simulink model "Sim_Induct_Harmon"  (R2019a)
settings: Solver=FixedStepAuto  StartTime=0.0  StopTime=sim_time  FixedStep=1e-6  MaxStep=1e-4  RelTol=1e-3
values from neighbouring files (symbols this model uses):
  J = 0.0025    [motor_parameters.mat]
  Laq = 0.001    [motor_parameters.mat]
  Lse = 0.001    [motor_parameters.mat]
  Ra = 2.08    [motor_parameters.mat]
  Rse = 5.7    [motor_parameters.mat]
  SEIP4 = [-14.225 -12.275 -10.725 -9.725 -9.1 -8.6 -8.075 -7.65 -7.2 -6.85 -6.492 -6.135 ... (45 elements, 1x45)]    [motor_parameters.mat]
  SEVP4 = [-160 -155 -150 -145 -140 -135 -130 -125 -120 -115 -110 -105 ... (45 elements, 1x45)]    [motor_parameters.mat]
  sim_off = sim_on    [double_load.m]    (also in fourfold_load.m; individual_load.m; triple_load.m)
  sim_on = 50*ones(1,28)    [double_load.m]    (also in fourfold_load.m; individual_load.m; triple_load.m)
  wm0 = 0    [motor_parameters.mat]
  wmo = 157.079632679    [motor_parameters.mat]
undefined symbols (not defined in the file or in its folder): C21, C22, C23, C24, L41, L42, L43, L44, L61, L62, L63, L64, R, R21, R22, R23, R24, R31, R32, R33, R34, R41, R42, R43, R44, R51, R52, R53, R54, R61, R62, R63, R64, R71, R72, R73, R74, Valpha5, Valpha6
libraries: powerlib x225, simulink x72
(part 2 of 3)

== system Sim_Induct_Harmon/ON_OFF_26 ==
  Clock8 : Clock
  Compare To Constant5 : simulink/Logic and Bit Operations/Compare To Constant  relop=>=  const=sim_on(26)  OutDataTypeStr=boolean
  Compare To Constat6 : simulink/Logic and Bit Operations/Compare To Constant  relop=<=  const=sim_off(26)  OutDataTypeStr=boolean
  OFF5 : powerlib/Power Electronics/Ideal Switch  Ron=0.001  Lon=0  IC=0  Rs=1e5  Cs=inf  Measurements=off
      settings: SourceProductName=Simscape Electrical
  ON5 : powerlib/Power Electronics/Ideal Switch  Ron=0.001  Lon=0  IC=0  Rs=1e5  Cs=inf  Measurements=off
      settings: SourceProductName=Simscape Electrical
  Conn1 : PMIOPort  Side=Left
  Conn2 : PMIOPort  Port=2  Side=Right
  wires:
  Clock8/1 -> Compare To Constat6/1, Compare To Constant5/1
  Compare To Constat6/1 -> OFF5/1
  Compare To Constant5/1 -> ON5/1
  connections:
  ON5/RConn1 -- OFF5/LConn1
  OFF5/RConn1 -- Conn2/RConn1
  ON5/LConn1 -- Conn1/RConn1

== system Sim_Induct_Harmon/ON_OFF_27 ==
  Clock8 : Clock
  Compare To Constant5 : simulink/Logic and Bit Operations/Compare To Constant  relop=>=  const=sim_on(27)  OutDataTypeStr=boolean
  Compare To Constat6 : simulink/Logic and Bit Operations/Compare To Constant  relop=<=  const=sim_off(27)  OutDataTypeStr=boolean
  OFF5 : powerlib/Power Electronics/Ideal Switch  Ron=0.001  Lon=0  IC=0  Rs=1e5  Cs=inf  Measurements=off
      settings: SourceProductName=Simscape Electrical
  ON5 : powerlib/Power Electronics/Ideal Switch  Ron=0.001  Lon=0  IC=0  Rs=1e5  Cs=inf  Measurements=off
      settings: SourceProductName=Simscape Electrical
  Conn1 : PMIOPort  Side=Left
  Conn2 : PMIOPort  Port=2  Side=Right
  wires:
  Clock8/1 -> Compare To Constat6/1, Compare To Constant5/1
  Compare To Constat6/1 -> OFF5/1
  Compare To Constant5/1 -> ON5/1
  connections:
  ON5/RConn1 -- OFF5/LConn1
  OFF5/RConn1 -- Conn2/RConn1
  ON5/LConn1 -- Conn1/RConn1

== system Sim_Induct_Harmon/ON_OFF_28 ==
  Clock8 : Clock
  Compare To Constant5 : simulink/Logic and Bit Operations/Compare To Constant  relop=>=  const=sim_on(28)  OutDataTypeStr=boolean
  Compare To Constat6 : simulink/Logic and Bit Operations/Compare To Constant  relop=<=  const=sim_off(28)  OutDataTypeStr=boolean
  OFF5 : powerlib/Power Electronics/Ideal Switch  Ron=0.001  Lon=0  IC=0  Rs=1e5  Cs=inf  Measurements=off
      settings: SourceProductName=Simscape Electrical
  ON5 : powerlib/Power Electronics/Ideal Switch  Ron=0.001  Lon=0  IC=0  Rs=1e5  Cs=inf  Measurements=off
      settings: SourceProductName=Simscape Electrical
  Conn1 : PMIOPort  Side=Left
  Conn2 : PMIOPort  Port=2  Side=Right
  wires:
  Clock8/1 -> Compare To Constat6/1, Compare To Constant5/1
  Compare To Constat6/1 -> OFF5/1
  Compare To Constant5/1 -> ON5/1
  connections:
  ON5/RConn1 -- OFF5/LConn1
  OFF5/RConn1 -- Conn2/RConn1
  ON5/LConn1 -- Conn1/RConn1

== system Sim_Induct_Harmon/ON_OFF_3 ==
  Clock1 : Clock
  Clock2 : Clock
  Clock3 : Clock
  Compare To Constant : simulink/Logic and Bit Operations/Compare To Constant  relop=>=  const=sim_on(3)  OutDataTypeStr=boolean
  Compare To Constant1 : simulink/Logic and Bit Operations/Compare To Constant  relop=>=  const=sim_off(3)  OutDataTypeStr=boolean
  Compare To Constant2 : simulink/Logic and Bit Operations/Compare To Constant  relop=>=  const=sim_on(3)  OutDataTypeStr=boolean
  Constant : Constant  Value=0
  Constant1 : Constant  Value=0
  Ideal Switch : powerlib/Power Electronics/Ideal Switch  Ron=0.001  Lon=0  IC=0  Rs=1e5  Cs=inf  Measurements=off
      settings: SourceProductName=Simscape Electrical
  Switch : Switch
  Switch1 : Switch
  Conn1 : PMIOPort  Side=Left
  Conn2 : PMIOPort  Port=2  Side=Left
  tag scope: tensao_3=global
  wires:
  Switch1/1 -> [tensao_3]
  Constant/1 -> Switch/3
  Switch/1 -> Switch1/3
  Clock1/1 -> Compare To Constant/1
  Clock2/1 -> Compare To Constant1/1
  Compare To Constant1/1 -> Switch1/2
  [fonte_tensao] -> Switch/1
  Constant1/1 -> Switch1/1
  Compare To Constant/1 -> Switch/2
  Clock3/1 -> Compare To Constant2/1
  Compare To Constant2/1 -> Ideal Switch/1
  connections:
  Conn1/RConn1 -- Ideal Switch/LConn1
  Ideal Switch/RConn1 -- Conn2/RConn1

== system Sim_Induct_Harmon/ON_OFF_4 ==
  Clock1 : Clock
  Clock2 : Clock
  Clock3 : Clock
  Compare To Constant : simulink/Logic and Bit Operations/Compare To Constant  relop=>=  const=sim_on(4)  OutDataTypeStr=boolean
  Compare To Constant1 : simulink/Logic and Bit Operations/Compare To Constant  relop=>=  const=sim_off(4)  OutDataTypeStr=boolean
  Compare To Constant2 : simulink/Logic and Bit Operations/Compare To Constant  relop=>=  const=sim_on(4)  OutDataTypeStr=boolean
  Constant : Constant  Value=0
  Constant1 : Constant  Value=0
  Ideal Switch : powerlib/Power Electronics/Ideal Switch  Ron=0.001  Lon=0  IC=0  Rs=1e5  Cs=inf  Measurements=off
      settings: SourceProductName=Simscape Electrical
  Switch : Switch
  Switch1 : Switch
  Conn1 : PMIOPort  Side=Left
  Conn2 : PMIOPort  Port=2  Side=Left
  tag scope: tensao_4=global
  wires:
  Switch1/1 -> [tensao_4]
  Constant/1 -> Switch/3
  Switch/1 -> Switch1/3
  Clock1/1 -> Compare To Constant/1
  Clock2/1 -> Compare To Constant1/1
  Compare To Constant1/1 -> Switch1/2
  [fonte_tensao] -> Switch/1
  Constant1/1 -> Switch1/1
  Compare To Constant/1 -> Switch/2
  Clock3/1 -> Compare To Constant2/1
  Compare To Constant2/1 -> Ideal Switch/1
  connections:
  Conn1/RConn1 -- Ideal Switch/LConn1
  Ideal Switch/RConn1 -- Conn2/RConn1

== system Sim_Induct_Harmon/ON_OFF_5 ==
  Clock1 : Clock
  Compare To Constant1 : simulink/Logic and Bit Operations/Compare To Constant  relop=>=  const=sim_on(5)  OutDataTypeStr=boolean
  Compare To Constat1 : simulink/Logic and Bit Operations/Compare To Constant  relop=<=  const=sim_off(5)  OutDataTypeStr=boolean
  OFF1 : powerlib/Power Electronics/Ideal Switch  Ron=0.001  Lon=0  IC=0  Rs=1e5  Cs=inf  Measurements=off
      settings: SourceProductName=Simscape Electrical
  ON1 : powerlib/Power Electronics/Ideal Switch  Ron=0.001  Lon=0  IC=0  Rs=1e5  Cs=inf  Measurements=off
      settings: SourceProductName=Simscape Electrical
  Conn1 : PMIOPort  Side=Left
  Conn2 : PMIOPort  Port=2  Side=Right
  wires:
  Compare To Constat1/1 -> OFF1/1
  Compare To Constant1/1 -> ON1/1
  Clock1/1 -> Compare To Constat1/1, Compare To Constant1/1
  connections:
  ON1/RConn1 -- OFF1/LConn1
  Conn1/RConn1 -- ON1/LConn1
  OFF1/RConn1 -- Conn2/RConn1

== system Sim_Induct_Harmon/ON_OFF_6 ==
  Clock1 : Clock
  Compare To Constant1 : simulink/Logic and Bit Operations/Compare To Constant  relop=>=  const=sim_on(6)  OutDataTypeStr=boolean
  Compare To Constat1 : simulink/Logic and Bit Operations/Compare To Constant  relop=<=  const=sim_off(6)  OutDataTypeStr=boolean
  OFF1 : powerlib/Power Electronics/Ideal Switch  Ron=0.001  Lon=0  IC=0  Rs=1e5  Cs=inf  Measurements=off
      settings: SourceProductName=Simscape Electrical
  ON1 : powerlib/Power Electronics/Ideal Switch  Ron=0.001  Lon=0  IC=0  Rs=1e5  Cs=inf  Measurements=off
      settings: SourceProductName=Simscape Electrical
  Conn1 : PMIOPort  Side=Left
  Conn2 : PMIOPort  Port=2  Side=Right
  wires:
  Compare To Constat1/1 -> OFF1/1
  Compare To Constant1/1 -> ON1/1
  Clock1/1 -> Compare To Constat1/1, Compare To Constant1/1
  connections:
  ON1/RConn1 -- OFF1/LConn1
  Conn1/RConn1 -- ON1/LConn1
  OFF1/RConn1 -- Conn2/RConn1

== system Sim_Induct_Harmon/ON_OFF_7 ==
  Clock1 : Clock
  Compare To Constant1 : simulink/Logic and Bit Operations/Compare To Constant  relop=>=  const=sim_on(7)  OutDataTypeStr=boolean
  Compare To Constat1 : simulink/Logic and Bit Operations/Compare To Constant  relop=<=  const=sim_off(7)  OutDataTypeStr=boolean
  OFF1 : powerlib/Power Electronics/Ideal Switch  Ron=0.001  Lon=0  IC=0  Rs=1e5  Cs=inf  Measurements=off
      settings: SourceProductName=Simscape Electrical
  ON1 : powerlib/Power Electronics/Ideal Switch  Ron=0.001  Lon=0  IC=0  Rs=1e5  Cs=inf  Measurements=off
      settings: SourceProductName=Simscape Electrical
  Conn1 : PMIOPort  Side=Left
  Conn2 : PMIOPort  Port=2  Side=Right
  wires:
  Compare To Constat1/1 -> OFF1/1
  Compare To Constant1/1 -> ON1/1
  Clock1/1 -> Compare To Constat1/1, Compare To Constant1/1
  connections:
  ON1/RConn1 -- OFF1/LConn1
  Conn1/RConn1 -- ON1/LConn1
  OFF1/RConn1 -- Conn2/RConn1

== system Sim_Induct_Harmon/ON_OFF_8 ==
  Clock1 : Clock
  Compare To Constant1 : simulink/Logic and Bit Operations/Compare To Constant  relop=>=  const=sim_on(8)  OutDataTypeStr=boolean
  Compare To Constat1 : simulink/Logic and Bit Operations/Compare To Constant  relop=<=  const=sim_off(8)  OutDataTypeStr=boolean
  OFF1 : powerlib/Power Electronics/Ideal Switch  Ron=0.001  Lon=0  IC=0  Rs=1e5  Cs=inf  Measurements=off
      settings: SourceProductName=Simscape Electrical
  ON1 : powerlib/Power Electronics/Ideal Switch  Ron=0.001  Lon=0  IC=0  Rs=1e5  Cs=inf  Measurements=off
      settings: SourceProductName=Simscape Electrical
  Conn1 : PMIOPort  Side=Left
  Conn2 : PMIOPort  Port=2  Side=Right
  wires:
  Compare To Constat1/1 -> OFF1/1
  Compare To Constant1/1 -> ON1/1
  Clock1/1 -> Compare To Constat1/1, Compare To Constant1/1
  connections:
  ON1/RConn1 -- OFF1/LConn1
  Conn1/RConn1 -- ON1/LConn1
  OFF1/RConn1 -- Conn2/RConn1

== system Sim_Induct_Harmon/ON_OFF_9 ==
  Clock4 : Clock
  Compare To Constant2 : simulink/Logic and Bit Operations/Compare To Constant  relop=>=  const=sim_on(9)  OutDataTypeStr=boolean
  Compare To Constat3 : simulink/Logic and Bit Operations/Compare To Constant  relop=<=  const=sim_off(9)  OutDataTypeStr=boolean
  OFF2 : powerlib/Power Electronics/Ideal Switch  Ron=0.001  Lon=0  IC=0  Rs=1e5  Cs=inf  Measurements=off
      settings: SourceProductName=Simscape Electrical
  ON2 : powerlib/Power Electronics/Ideal Switch  Ron=0.001  Lon=0  IC=0  Rs=1e5  Cs=inf  Measurements=off
      settings: SourceProductName=Simscape Electrical
  Conn1 : PMIOPort  Side=Left
  Conn2 : PMIOPort  Port=2  Side=Right
  wires:
  Compare To Constant2/1 -> ON2/1
  Compare To Constat3/1 -> OFF2/1
  Clock4/1 -> Compare To Constat3/1, Compare To Constant2/1
  connections:
  OFF2/RConn1 -- Conn2/RConn1
  ON2/RConn1 -- OFF2/LConn1
  ON2/LConn1 -- Conn1/RConn1

== system Sim_Induct_Harmon/RL_1 ==
  note: LOAD
  Scope : Scope
  Scope1 : Scope
  Series RLC Branch : powerlib/Elements/Series RLC Branch  LConnTagsString=__new0  RConnTagsString=__new0  BranchType=R  Resistance=R41  Inductance=1e-3  SetiL0=off  InitialCurrent=0  Capacitance=1e-6  Setx0=off  InitialVoltage=0  Measurements=None
      settings: SourceProductName=Simscape Electrical
  Series RLC Branch1 : powerlib/Elements/Series RLC Branch  LConnTagsString=__new0  RConnTagsString=__new0  BranchType=L  Resistance=1  Inductance=L41  SetiL0=off  InitialCurrent=0  Capacitance=1e-6  Setx0=off  InitialVoltage=0  Measurements=None
      settings: SourceProductName=Simscape Electrical
  To Workspace1 : ToWorkspace  VariableName=corrente_rl_1  SampleTime=-1
  To Workspace4 : ToWorkspace  VariableName=tensao_rl_1  SampleTime=-1
  V_Load : powerlib/Measurements/Voltage Measurement  PhasorSimulation=off  OutputType=Complex  PSBequivalent=0
      settings: SourceProductName=Simscape Electrical
  i_Load : powerlib/Measurements/Current Measurement  Tag=PoWeRsYsTeMmEaSuReMeNt  PhasorSimulation=off  OutputType=Magnitude  PSBequivalent=0
      settings: SourceProductName=Simscape Electrical
  Conn1 : PMIOPort  Side=Left
  Conn2 : PMIOPort  Port=2  Side=Left
  wires:
  V_Load/1 -> To Workspace4/1, Scope/1
  i_Load/1 -> To Workspace1/1, Scope1/1
  connections:
  Series RLC Branch/LConn1 -- V_Load/LConn1 -- i_Load/RConn1
  Conn1/RConn1 -- i_Load/LConn1
  V_Load/LConn2 -- Conn2/RConn1 -- Series RLC Branch1/RConn1
  Series RLC Branch1/LConn1 -- Series RLC Branch/RConn1

== system Sim_Induct_Harmon/RL_2 ==
  note: LOAD
  Scope : Scope
  Scope1 : Scope
  Series RLC Branch : powerlib/Elements/Series RLC Branch  LConnTagsString=__new0  RConnTagsString=__new0  BranchType=R  Resistance=R42  Inductance=1e-3  SetiL0=off  InitialCurrent=0  Capacitance=1e-6  Setx0=off  InitialVoltage=0  Measurements=None
      settings: SourceProductName=Simscape Electrical
  Series RLC Branch1 : powerlib/Elements/Series RLC Branch  LConnTagsString=__new0  RConnTagsString=__new0  BranchType=L  Resistance=1  Inductance=L42  SetiL0=off  InitialCurrent=0  Capacitance=1e-6  Setx0=off  InitialVoltage=0  Measurements=None
      settings: SourceProductName=Simscape Electrical
  To Workspace1 : ToWorkspace  VariableName=corrente_rl_2  SampleTime=-1
  To Workspace4 : ToWorkspace  VariableName=tensao_rl_2  SampleTime=-1
  V_Load : powerlib/Measurements/Voltage Measurement  PhasorSimulation=off  OutputType=Complex  PSBequivalent=0
      settings: SourceProductName=Simscape Electrical
  i_Load : powerlib/Measurements/Current Measurement  Tag=PoWeRsYsTeMmEaSuReMeNt  PhasorSimulation=off  OutputType=Magnitude  PSBequivalent=0
      settings: SourceProductName=Simscape Electrical
  Conn1 : PMIOPort  Side=Left
  Conn2 : PMIOPort  Port=2  Side=Left
  wires:
  V_Load/1 -> To Workspace4/1, Scope/1
  i_Load/1 -> To Workspace1/1, Scope1/1
  connections:
  Series RLC Branch/LConn1 -- V_Load/LConn1 -- i_Load/RConn1
  Conn1/RConn1 -- i_Load/LConn1
  V_Load/LConn2 -- Conn2/RConn1 -- Series RLC Branch1/RConn1
  Series RLC Branch1/LConn1 -- Series RLC Branch/RConn1

== system Sim_Induct_Harmon/RL_3 ==
  note: LOAD
  Scope : Scope
  Scope1 : Scope
  Series RLC Branch : powerlib/Elements/Series RLC Branch  LConnTagsString=__new0  RConnTagsString=__new0  BranchType=R  Resistance=R43  Inductance=1e-3  SetiL0=off  InitialCurrent=0  Capacitance=1e-6  Setx0=off  InitialVoltage=0  Measurements=None
      settings: SourceProductName=Simscape Electrical
  Series RLC Branch1 : powerlib/Elements/Series RLC Branch  LConnTagsString=__new0  RConnTagsString=__new0  BranchType=L  Resistance=1  Inductance=L43  SetiL0=off  InitialCurrent=0  Capacitance=1e-6  Setx0=off  InitialVoltage=0  Measurements=None
      settings: SourceProductName=Simscape Electrical
  To Workspace1 : ToWorkspace  VariableName=corrente_rl_3  SampleTime=-1
  To Workspace4 : ToWorkspace  VariableName=tensao_rl_3  SampleTime=-1
  V_Load : powerlib/Measurements/Voltage Measurement  PhasorSimulation=off  OutputType=Complex  PSBequivalent=0
      settings: SourceProductName=Simscape Electrical
  i_Load : powerlib/Measurements/Current Measurement  Tag=PoWeRsYsTeMmEaSuReMeNt  PhasorSimulation=off  OutputType=Magnitude  PSBequivalent=0
      settings: SourceProductName=Simscape Electrical
  Conn1 : PMIOPort  Side=Left
  Conn2 : PMIOPort  Port=2  Side=Left
  wires:
  V_Load/1 -> To Workspace4/1, Scope/1
  i_Load/1 -> To Workspace1/1, Scope1/1
  connections:
  Series RLC Branch/LConn1 -- V_Load/LConn1 -- i_Load/RConn1
  Conn1/RConn1 -- i_Load/LConn1
  V_Load/LConn2 -- Conn2/RConn1 -- Series RLC Branch1/RConn1
  Series RLC Branch1/LConn1 -- Series RLC Branch/RConn1

== system Sim_Induct_Harmon/RL_4 ==
  note: LOAD
  Scope : Scope
  Scope1 : Scope
  Series RLC Branch : powerlib/Elements/Series RLC Branch  LConnTagsString=__new0  RConnTagsString=__new0  BranchType=R  Resistance=R44  Inductance=1e-3  SetiL0=off  InitialCurrent=0  Capacitance=1e-6  Setx0=off  InitialVoltage=0  Measurements=None
      settings: SourceProductName=Simscape Electrical
  Series RLC Branch1 : powerlib/Elements/Series RLC Branch  LConnTagsString=__new0  RConnTagsString=__new0  BranchType=L  Resistance=1  Inductance=L44  SetiL0=off  InitialCurrent=0  Capacitance=1e-6  Setx0=off  InitialVoltage=0  Measurements=None
      settings: SourceProductName=Simscape Electrical
  To Workspace1 : ToWorkspace  VariableName=corrente_rl_4  SampleTime=-1
  To Workspace4 : ToWorkspace  VariableName=tensao_rl_4  SampleTime=-1
  V_Load : powerlib/Measurements/Voltage Measurement  PhasorSimulation=off  OutputType=Complex  PSBequivalent=0
      settings: SourceProductName=Simscape Electrical
  i_Load : powerlib/Measurements/Current Measurement  Tag=PoWeRsYsTeMmEaSuReMeNt  PhasorSimulation=off  OutputType=Magnitude  PSBequivalent=0
      settings: SourceProductName=Simscape Electrical
  Conn1 : PMIOPort  Side=Left
  Conn2 : PMIOPort  Port=2  Side=Left
  wires:
  V_Load/1 -> To Workspace4/1, Scope/1
  i_Load/1 -> To Workspace1/1, Scope1/1
  connections:
  Series RLC Branch/LConn1 -- V_Load/LConn1 -- i_Load/RConn1
  Conn1/RConn1 -- i_Load/LConn1
  V_Load/LConn2 -- Conn2/RConn1 -- Series RLC Branch1/RConn1
  Series RLC Branch1/LConn1 -- Series RLC Branch/RConn1

== system Sim_Induct_Harmon/R_1 ==
  note: LOAD
  Scope : Scope
  Scope1 : Scope
  Series RLC Branch : powerlib/Elements/Series RLC Branch  LConnTagsString=__new0  RConnTagsString=__new0  BranchType=R  Resistance=R31  Inductance=1e-3  SetiL0=off  InitialCurrent=0  Capacitance=1e-6  Setx0=off  InitialVoltage=0  Measurements=None
      settings: SourceProductName=Simscape Electrical
  To Workspace1 : ToWorkspace  VariableName=corrente_r_1  SampleTime=-1
  To Workspace4 : ToWorkspace  VariableName=tensao_r_1  SampleTime=-1
  V_Load : powerlib/Measurements/Voltage Measurement  PhasorSimulation=off  OutputType=Complex  PSBequivalent=0
      settings: SourceProductName=Simscape Electrical
  i_Load : powerlib/Measurements/Current Measurement  Tag=PoWeRsYsTeMmEaSuReMeNt  PhasorSimulation=off  OutputType=Magnitude  PSBequivalent=0
      settings: SourceProductName=Simscape Electrical
  Conn1 : PMIOPort  Side=Left
  Conn2 : PMIOPort  Port=2  Side=Left
  wires:
  V_Load/1 -> To Workspace4/1, Scope/1
  i_Load/1 -> To Workspace1/1, Scope1/1
  connections:
  Series RLC Branch/LConn1 -- V_Load/LConn1 -- i_Load/RConn1
  Series RLC Branch/RConn1 -- V_Load/LConn2 -- Conn2/RConn1
  Conn1/RConn1 -- i_Load/LConn1

== system Sim_Induct_Harmon/R_2 ==
  note: LOAD
  Scope : Scope
  Scope1 : Scope
  Series RLC Branch : powerlib/Elements/Series RLC Branch  LConnTagsString=__new0  RConnTagsString=__new0  BranchType=R  Resistance=R32  Inductance=1e-3  SetiL0=off  InitialCurrent=0  Capacitance=1e-6  Setx0=off  InitialVoltage=0  Measurements=None
      settings: SourceProductName=Simscape Electrical
  To Workspace1 : ToWorkspace  VariableName=corrente_r_2  SampleTime=-1
  To Workspace4 : ToWorkspace  VariableName=tensao_r_2  SampleTime=-1
  V_Load : powerlib/Measurements/Voltage Measurement  PhasorSimulation=off  OutputType=Complex  PSBequivalent=0
      settings: SourceProductName=Simscape Electrical
  i_Load : powerlib/Measurements/Current Measurement  Tag=PoWeRsYsTeMmEaSuReMeNt  PhasorSimulation=off  OutputType=Magnitude  PSBequivalent=0
      settings: SourceProductName=Simscape Electrical
  Conn1 : PMIOPort  Side=Left
  Conn2 : PMIOPort  Port=2  Side=Left
  wires:
  V_Load/1 -> To Workspace4/1, Scope/1
  i_Load/1 -> To Workspace1/1, Scope1/1
  connections:
  Series RLC Branch/LConn1 -- V_Load/LConn1 -- i_Load/RConn1
  Series RLC Branch/RConn1 -- V_Load/LConn2 -- Conn2/RConn1
  Conn1/RConn1 -- i_Load/LConn1

== system Sim_Induct_Harmon/R_3 ==
  note: LOAD
  Scope : Scope
  Scope1 : Scope
  Series RLC Branch : powerlib/Elements/Series RLC Branch  LConnTagsString=__new0  RConnTagsString=__new0  BranchType=R  Resistance=R33  Inductance=1e-3  SetiL0=off  InitialCurrent=0  Capacitance=1e-6  Setx0=off  InitialVoltage=0  Measurements=None
      settings: SourceProductName=Simscape Electrical
  To Workspace1 : ToWorkspace  VariableName=corrente_r_3  SampleTime=-1
  To Workspace4 : ToWorkspace  VariableName=tensao_r_3  SampleTime=-1
  V_Load : powerlib/Measurements/Voltage Measurement  PhasorSimulation=off  OutputType=Complex  PSBequivalent=0
      settings: SourceProductName=Simscape Electrical
  i_Load : powerlib/Measurements/Current Measurement  Tag=PoWeRsYsTeMmEaSuReMeNt  PhasorSimulation=off  OutputType=Magnitude  PSBequivalent=0
      settings: SourceProductName=Simscape Electrical
  Conn1 : PMIOPort  Side=Left
  Conn2 : PMIOPort  Port=2  Side=Left
  wires:
  V_Load/1 -> To Workspace4/1, Scope/1
  i_Load/1 -> To Workspace1/1, Scope1/1
  connections:
  Series RLC Branch/LConn1 -- V_Load/LConn1 -- i_Load/RConn1
  Series RLC Branch/RConn1 -- V_Load/LConn2 -- Conn2/RConn1
  Conn1/RConn1 -- i_Load/LConn1

== system Sim_Induct_Harmon/R_4 ==
  note: LOAD
  Scope : Scope
  Scope1 : Scope
  Series RLC Branch : powerlib/Elements/Series RLC Branch  LConnTagsString=__new0  RConnTagsString=__new0  BranchType=R  Resistance=R34  Inductance=1e-3  SetiL0=off  InitialCurrent=0  Capacitance=1e-6  Setx0=off  InitialVoltage=0  Measurements=None
      settings: SourceProductName=Simscape Electrical
  To Workspace1 : ToWorkspace  VariableName=corrente_r_4  SampleTime=-1
  To Workspace4 : ToWorkspace  VariableName=tensao_r_4  SampleTime=-1
  V_Load : powerlib/Measurements/Voltage Measurement  PhasorSimulation=off  OutputType=Complex  PSBequivalent=0
      settings: SourceProductName=Simscape Electrical
  i_Load : powerlib/Measurements/Current Measurement  Tag=PoWeRsYsTeMmEaSuReMeNt  PhasorSimulation=off  OutputType=Magnitude  PSBequivalent=0
      settings: SourceProductName=Simscape Electrical
  Conn1 : PMIOPort  Side=Left
  Conn2 : PMIOPort  Port=2  Side=Left
  wires:
  V_Load/1 -> To Workspace4/1, Scope/1
  i_Load/1 -> To Workspace1/1, Scope1/1
  connections:
  Series RLC Branch/LConn1 -- V_Load/LConn1 -- i_Load/RConn1
  Series RLC Branch/RConn1 -- V_Load/LConn2 -- Conn2/RConn1
  Conn1/RConn1 -- i_Load/LConn1

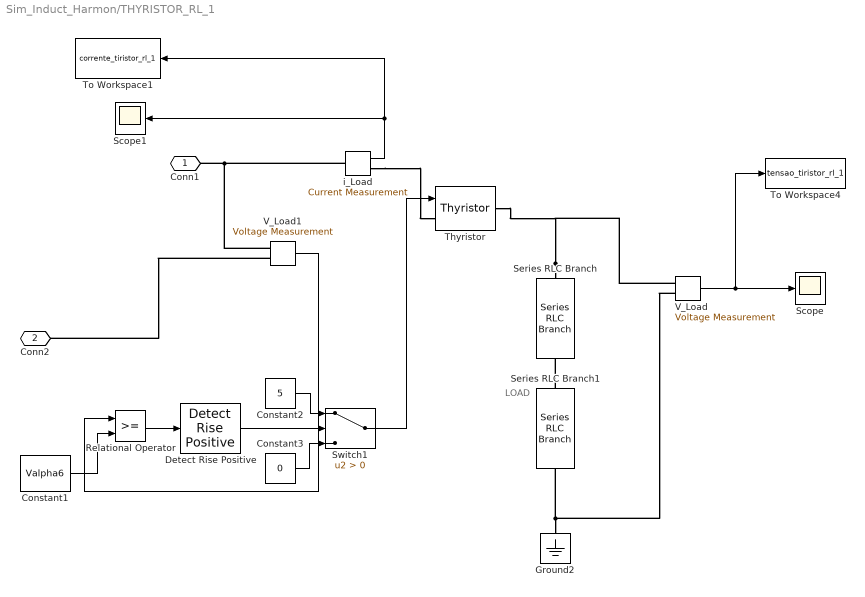
== system Sim_Induct_Harmon/THYRISTOR_RL_1 ==
  note: LOAD
  Constant1 : Constant  Value=Valpha6
  Constant2 : Constant  Value=5
  Constant3 : Constant  Value=0
  Detect Rise Positive : simulink/Logic and Bit Operations/Detect Rise Positive  vinit=0  OutDataTypeStr=boolean
  Ground2 : powerlib/Elements/Ground  LConnTagsString=a
      settings: SourceProductName=Simscape Electrical
  Relational Operator : RelationalOperator  OutDataTypeStr=boolean  RndMeth=Simplest
  Scope : Scope
  Scope1 : Scope
  Series RLC Branch : powerlib/Elements/Series RLC Branch  LConnTagsString=__new0  RConnTagsString=__new0  BranchType=R  Resistance=R61  Inductance=1e-3  SetiL0=off  InitialCurrent=0  Capacitance=1e-6  Setx0=off  InitialVoltage=0  Measurements=None
      settings: SourceProductName=Simscape Electrical
  Series RLC Branch1 : powerlib/Elements/Series RLC Branch  LConnTagsString=__new0  RConnTagsString=__new0  BranchType=L  Resistance=1  Inductance=L61  SetiL0=off  InitialCurrent=0  Capacitance=1e-6  Setx0=off  InitialVoltage=0  Measurements=None
      settings: SourceProductName=Simscape Electrical
  Switch1 : Switch  Criteria=u2 > Threshold
  Thyristor : powerlib/Power Electronics/Thyristor  Ron=0.001  Lon=0  Vf=0.8  IC=0  Rs=500  Cs=250e-9  Measurements=off
      settings: SourceProductName=Simscape Electrical
  To Workspace1 : ToWorkspace  VariableName=corrente_tiristor_rl_1  SampleTime=-1
  To Workspace4 : ToWorkspace  VariableName=tensao_tiristor_rl_1  SampleTime=-1
  V_Load : powerlib/Measurements/Voltage Measurement  PhasorSimulation=off  OutputType=Complex  PSBequivalent=0
      settings: SourceProductName=Simscape Electrical
  V_Load1 : powerlib/Measurements/Voltage Measurement  PhasorSimulation=off  OutputType=Complex  PSBequivalent=0
      settings: SourceProductName=Simscape Electrical
  i_Load : powerlib/Measurements/Current Measurement  Tag=PoWeRsYsTeMmEaSuReMeNt  PhasorSimulation=off  OutputType=Magnitude  PSBequivalent=0
      settings: SourceProductName=Simscape Electrical
  Conn1 : PMIOPort  Side=Left
  Conn2 : PMIOPort  Port=2  Side=Left
  wires:
  V_Load1/1 -> Relational Operator/1
  Constant1/1 -> Relational Operator/2
  Detect Rise Positive/1 -> Switch1/2
  Constant3/1 -> Switch1/3
  Relational Operator/1 -> Detect Rise Positive/1
  Constant2/1 -> Switch1/1
  i_Load/1 -> To Workspace1/1, Scope1/1
  V_Load/1 -> To Workspace4/1, Scope/1
  Switch1/1 -> Thyristor/1
  connections:
  Series RLC Branch1/LConn1 -- Series RLC Branch/RConn1
  Series RLC Branch/LConn1 -- V_Load/LConn1 -- Thyristor/RConn1
  V_Load/LConn2 -- Ground2/LConn1 -- Series RLC Branch1/RConn1
  i_Load/RConn1 -- Thyristor/LConn1
  V_Load1/LConn1 -- i_Load/LConn1 -- Conn1/RConn1
  V_Load1/LConn2 -- Conn2/RConn1

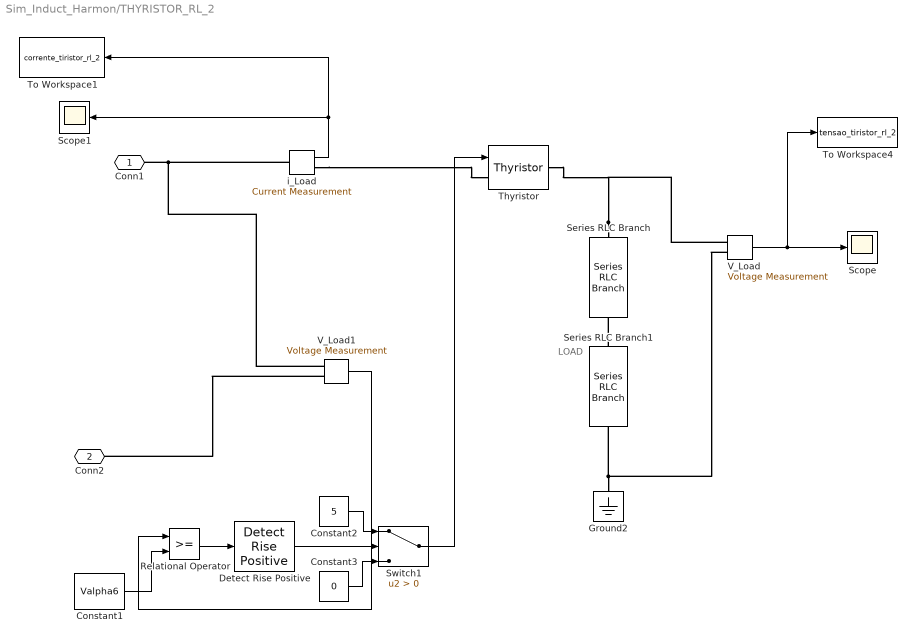
== system Sim_Induct_Harmon/THYRISTOR_RL_2 ==
  note: LOAD
  Constant1 : Constant  Value=Valpha6
  Constant2 : Constant  Value=5
  Constant3 : Constant  Value=0
  Detect Rise Positive : simulink/Logic and Bit Operations/Detect Rise Positive  vinit=0  OutDataTypeStr=boolean
  Ground2 : powerlib/Elements/Ground  LConnTagsString=a
      settings: SourceProductName=Simscape Electrical
  Relational Operator : RelationalOperator  OutDataTypeStr=boolean  RndMeth=Simplest
  Scope : Scope
  Scope1 : Scope
  Series RLC Branch : powerlib/Elements/Series RLC Branch  LConnTagsString=__new0  RConnTagsString=__new0  BranchType=R  Resistance=R62  Inductance=1e-3  SetiL0=off  InitialCurrent=0  Capacitance=1e-6  Setx0=off  InitialVoltage=0  Measurements=None
      settings: SourceProductName=Simscape Electrical
  Series RLC Branch1 : powerlib/Elements/Series RLC Branch  LConnTagsString=__new0  RConnTagsString=__new0  BranchType=L  Resistance=1  Inductance=L62  SetiL0=off  InitialCurrent=0  Capacitance=1e-6  Setx0=off  InitialVoltage=0  Measurements=None
      settings: SourceProductName=Simscape Electrical
  Switch1 : Switch  Criteria=u2 > Threshold
  Thyristor : powerlib/Power Electronics/Thyristor  Ron=0.001  Lon=0  Vf=0.8  IC=0  Rs=500  Cs=250e-9  Measurements=off
      settings: SourceProductName=Simscape Electrical
  To Workspace1 : ToWorkspace  VariableName=corrente_tiristor_rl_2  SampleTime=-1
  To Workspace4 : ToWorkspace  VariableName=tensao_tiristor_rl_2  SampleTime=-1
  V_Load : powerlib/Measurements/Voltage Measurement  PhasorSimulation=off  OutputType=Complex  PSBequivalent=0
      settings: SourceProductName=Simscape Electrical
  V_Load1 : powerlib/Measurements/Voltage Measurement  PhasorSimulation=off  OutputType=Complex  PSBequivalent=0
      settings: SourceProductName=Simscape Electrical
  i_Load : powerlib/Measurements/Current Measurement  Tag=PoWeRsYsTeMmEaSuReMeNt  PhasorSimulation=off  OutputType=Magnitude  PSBequivalent=0
      settings: SourceProductName=Simscape Electrical
  Conn1 : PMIOPort  Side=Left
  Conn2 : PMIOPort  Port=2  Side=Left
  wires:
  V_Load1/1 -> Relational Operator/1
  Constant1/1 -> Relational Operator/2
  Detect Rise Positive/1 -> Switch1/2
  Constant3/1 -> Switch1/3
  Relational Operator/1 -> Detect Rise Positive/1
  Constant2/1 -> Switch1/1
  i_Load/1 -> To Workspace1/1, Scope1/1
  V_Load/1 -> To Workspace4/1, Scope/1
  Switch1/1 -> Thyristor/1
  connections:
  Series RLC Branch1/LConn1 -- Series RLC Branch/RConn1
  Series RLC Branch/LConn1 -- V_Load/LConn1 -- Thyristor/RConn1
  V_Load/LConn2 -- Ground2/LConn1 -- Series RLC Branch1/RConn1
  i_Load/RConn1 -- Thyristor/LConn1
  V_Load1/LConn1 -- i_Load/LConn1 -- Conn1/RConn1
  V_Load1/LConn2 -- Conn2/RConn1

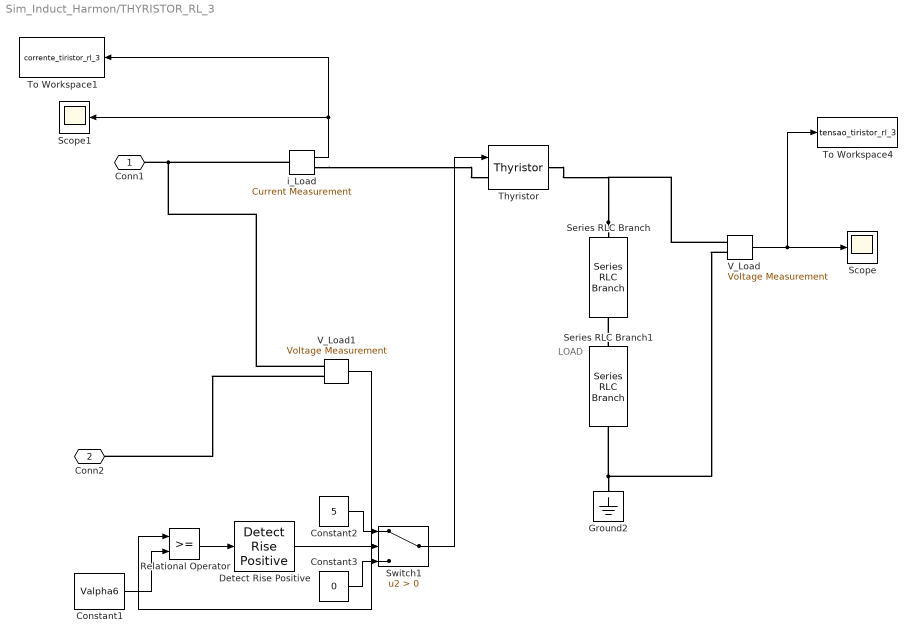
== system Sim_Induct_Harmon/THYRISTOR_RL_3 ==
  note: LOAD
  Constant1 : Constant  Value=Valpha6
  Constant2 : Constant  Value=5
  Constant3 : Constant  Value=0
  Detect Rise Positive : simulink/Logic and Bit Operations/Detect Rise Positive  vinit=0  OutDataTypeStr=boolean
  Ground2 : powerlib/Elements/Ground  LConnTagsString=a
      settings: SourceProductName=Simscape Electrical
  Relational Operator : RelationalOperator  OutDataTypeStr=boolean  RndMeth=Simplest
  Scope : Scope
  Scope1 : Scope
  Series RLC Branch : powerlib/Elements/Series RLC Branch  LConnTagsString=__new0  RConnTagsString=__new0  BranchType=R  Resistance=R63  Inductance=1e-3  SetiL0=off  InitialCurrent=0  Capacitance=1e-6  Setx0=off  InitialVoltage=0  Measurements=None
      settings: SourceProductName=Simscape Electrical
  Series RLC Branch1 : powerlib/Elements/Series RLC Branch  LConnTagsString=__new0  RConnTagsString=__new0  BranchType=L  Resistance=1  Inductance=L63  SetiL0=off  InitialCurrent=0  Capacitance=1e-6  Setx0=off  InitialVoltage=0  Measurements=None
      settings: SourceProductName=Simscape Electrical
  Switch1 : Switch  Criteria=u2 > Threshold
  Thyristor : powerlib/Power Electronics/Thyristor  Ron=0.001  Lon=0  Vf=0.8  IC=0  Rs=500  Cs=250e-9  Measurements=off
      settings: SourceProductName=Simscape Electrical
  To Workspace1 : ToWorkspace  VariableName=corrente_tiristor_rl_3  SampleTime=-1
  To Workspace4 : ToWorkspace  VariableName=tensao_tiristor_rl_3  SampleTime=-1
  V_Load : powerlib/Measurements/Voltage Measurement  PhasorSimulation=off  OutputType=Complex  PSBequivalent=0
      settings: SourceProductName=Simscape Electrical
  V_Load1 : powerlib/Measurements/Voltage Measurement  PhasorSimulation=off  OutputType=Complex  PSBequivalent=0
      settings: SourceProductName=Simscape Electrical
  i_Load : powerlib/Measurements/Current Measurement  Tag=PoWeRsYsTeMmEaSuReMeNt  PhasorSimulation=off  OutputType=Magnitude  PSBequivalent=0
      settings: SourceProductName=Simscape Electrical
  Conn1 : PMIOPort  Side=Left
  Conn2 : PMIOPort  Port=2  Side=Left
  wires:
  V_Load1/1 -> Relational Operator/1
  Constant1/1 -> Relational Operator/2
  Detect Rise Positive/1 -> Switch1/2
  Constant3/1 -> Switch1/3
  Relational Operator/1 -> Detect Rise Positive/1
  Constant2/1 -> Switch1/1
  i_Load/1 -> To Workspace1/1, Scope1/1
  V_Load/1 -> To Workspace4/1, Scope/1
  Switch1/1 -> Thyristor/1
  connections:
  Series RLC Branch1/LConn1 -- Series RLC Branch/RConn1
  Series RLC Branch/LConn1 -- V_Load/LConn1 -- Thyristor/RConn1
  V_Load/LConn2 -- Ground2/LConn1 -- Series RLC Branch1/RConn1
  i_Load/RConn1 -- Thyristor/LConn1
  V_Load1/LConn1 -- i_Load/LConn1 -- Conn1/RConn1
  V_Load1/LConn2 -- Conn2/RConn1

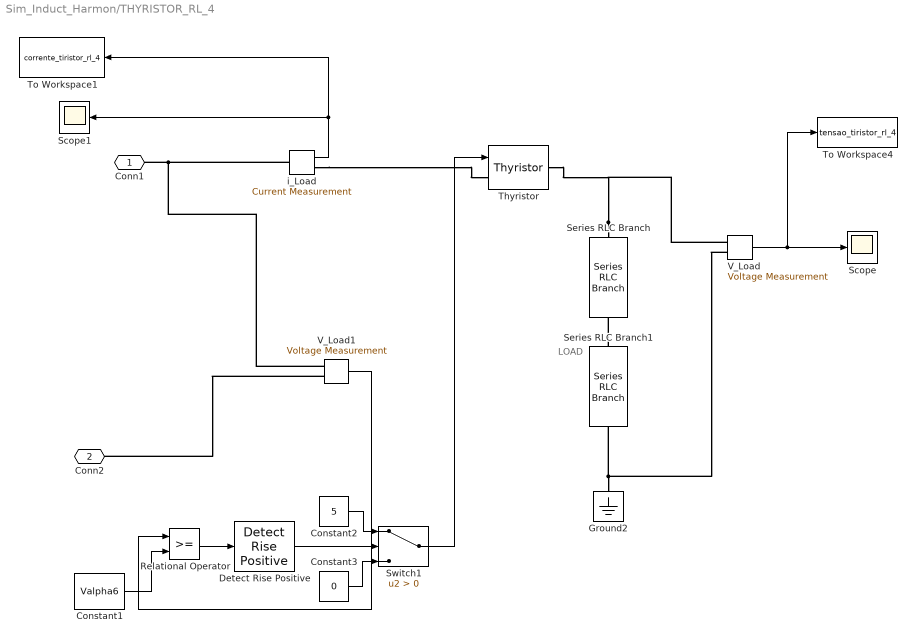
== system Sim_Induct_Harmon/THYRISTOR_RL_4 ==
  note: LOAD
  Constant1 : Constant  Value=Valpha6
  Constant2 : Constant  Value=5
  Constant3 : Constant  Value=0
  Detect Rise Positive : simulink/Logic and Bit Operations/Detect Rise Positive  vinit=0  OutDataTypeStr=boolean
  Ground2 : powerlib/Elements/Ground  LConnTagsString=a
      settings: SourceProductName=Simscape Electrical
  Relational Operator : RelationalOperator  OutDataTypeStr=boolean  RndMeth=Simplest
  Scope : Scope
  Scope1 : Scope
  Series RLC Branch : powerlib/Elements/Series RLC Branch  LConnTagsString=__new0  RConnTagsString=__new0  BranchType=R  Resistance=R64  Inductance=1e-3  SetiL0=off  InitialCurrent=0  Capacitance=1e-6  Setx0=off  InitialVoltage=0  Measurements=None
      settings: SourceProductName=Simscape Electrical
  Series RLC Branch1 : powerlib/Elements/Series RLC Branch  LConnTagsString=__new0  RConnTagsString=__new0  BranchType=L  Resistance=1  Inductance=L64  SetiL0=off  InitialCurrent=0  Capacitance=1e-6  Setx0=off  InitialVoltage=0  Measurements=None
      settings: SourceProductName=Simscape Electrical
  Switch1 : Switch  Criteria=u2 > Threshold
  Thyristor : powerlib/Power Electronics/Thyristor  Ron=0.001  Lon=0  Vf=0.8  IC=0  Rs=500  Cs=250e-9  Measurements=off
      settings: SourceProductName=Simscape Electrical
  To Workspace1 : ToWorkspace  VariableName=corrente_tiristor_rl_4  SampleTime=-1
  To Workspace4 : ToWorkspace  VariableName=tensao_tiristor_rl_4  SampleTime=-1
  V_Load : powerlib/Measurements/Voltage Measurement  PhasorSimulation=off  OutputType=Complex  PSBequivalent=0
      settings: SourceProductName=Simscape Electrical
  V_Load1 : powerlib/Measurements/Voltage Measurement  PhasorSimulation=off  OutputType=Complex  PSBequivalent=0
      settings: SourceProductName=Simscape Electrical
  i_Load : powerlib/Measurements/Current Measurement  Tag=PoWeRsYsTeMmEaSuReMeNt  PhasorSimulation=off  OutputType=Magnitude  PSBequivalent=0
      settings: SourceProductName=Simscape Electrical
  Conn1 : PMIOPort  Side=Left
  Conn2 : PMIOPort  Port=2  Side=Left
  wires:
  V_Load1/1 -> Relational Operator/1
  Constant1/1 -> Relational Operator/2
  Detect Rise Positive/1 -> Switch1/2
  Constant3/1 -> Switch1/3
  Relational Operator/1 -> Detect Rise Positive/1
  Constant2/1 -> Switch1/1
  i_Load/1 -> To Workspace1/1, Scope1/1
  V_Load/1 -> To Workspace4/1, Scope/1
  Switch1/1 -> Thyristor/1
  connections:
  Series RLC Branch1/LConn1 -- Series RLC Branch/RConn1
  Series RLC Branch/LConn1 -- V_Load/LConn1 -- Thyristor/RConn1
  V_Load/LConn2 -- Ground2/LConn1 -- Series RLC Branch1/RConn1
  i_Load/RConn1 -- Thyristor/LConn1
  V_Load1/LConn1 -- i_Load/LConn1 -- Conn1/RConn1
  V_Load1/LConn2 -- Conn2/RConn1

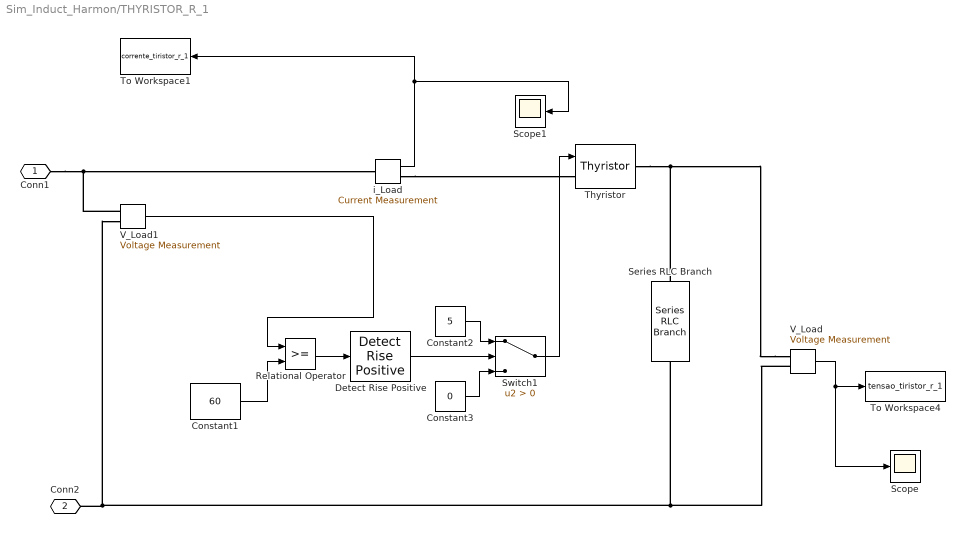
== system Sim_Induct_Harmon/THYRISTOR_R_1 ==
  Constant1 : Constant  Value=60
  Constant2 : Constant  Value=5
  Constant3 : Constant  Value=0
  Detect Rise Positive : simulink/Logic and Bit Operations/Detect Rise Positive  vinit=0  OutDataTypeStr=boolean
  Relational Operator : RelationalOperator  OutDataTypeStr=boolean  RndMeth=Simplest
  Scope : Scope
  Scope1 : Scope
  Series RLC Branch : powerlib/Elements/Series RLC Branch  LConnTagsString=__new0  RConnTagsString=__new0  BranchType=R  Resistance=R51  Inductance=1e-3  SetiL0=off  InitialCurrent=0  Capacitance=1e-6  Setx0=off  InitialVoltage=0  Measurements=None
      settings: SourceProductName=Simscape Electrical
  Switch1 : Switch  Criteria=u2 > Threshold
  Thyristor : powerlib/Power Electronics/Thyristor  Ron=0.001  Lon=0  Vf=0.8  IC=0  Rs=500  Cs=250e-9  Measurements=off
      settings: SourceProductName=Simscape Electrical
  To Workspace1 : ToWorkspace  VariableName=corrente_tiristor_r_1  SampleTime=-1
  To Workspace4 : ToWorkspace  VariableName=tensao_tiristor_r_1  SampleTime=-1
  V_Load : powerlib/Measurements/Voltage Measurement  PhasorSimulation=off  OutputType=Complex  PSBequivalent=0
      settings: SourceProductName=Simscape Electrical
  V_Load1 : powerlib/Measurements/Voltage Measurement  PhasorSimulation=off  OutputType=Complex  PSBequivalent=0
      settings: SourceProductName=Simscape Electrical
  i_Load : powerlib/Measurements/Current Measurement  Tag=PoWeRsYsTeMmEaSuReMeNt  PhasorSimulation=off  OutputType=Magnitude  PSBequivalent=0
      settings: SourceProductName=Simscape Electrical
  Conn1 : PMIOPort  Side=Left
  Conn2 : PMIOPort  Port=2  Side=Left
  wires:
  Constant3/1 -> Switch1/3
  Constant2/1 -> Switch1/1
  Constant1/1 -> Relational Operator/2
  Relational Operator/1 -> Detect Rise Positive/1
  i_Load/1 -> To Workspace1/1, Scope1/1
  Detect Rise Positive/1 -> Switch1/2
  V_Load1/1 -> Relational Operator/1
  V_Load/1 -> Scope/1, To Workspace4/1
  Switch1/1 -> Thyristor/1
  connections:
  V_Load/LConn1 -- Series RLC Branch/LConn1 -- Thyristor/RConn1
  Conn1/RConn1 -- V_Load1/LConn1 -- i_Load/LConn1
  i_Load/RConn1 -- Thyristor/LConn1
  V_Load/LConn2 -- Series RLC Branch/RConn1 -- Conn2/RConn1 -- V_Load1/LConn2

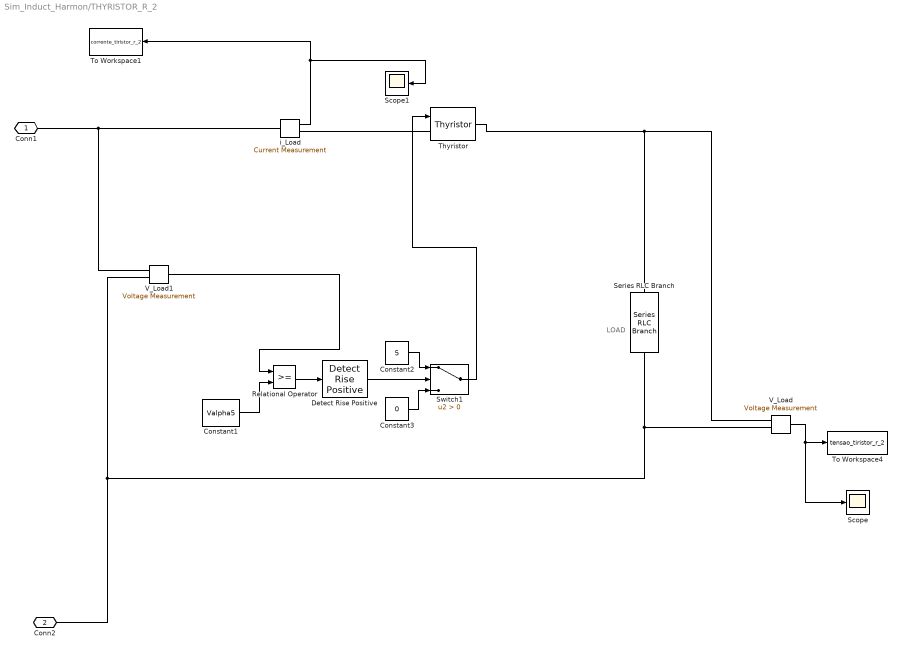
== system Sim_Induct_Harmon/THYRISTOR_R_2 ==
  note: LOAD
  Constant1 : Constant  Value=Valpha5
  Constant2 : Constant  Value=5
  Constant3 : Constant  Value=0
  Detect Rise Positive : simulink/Logic and Bit Operations/Detect Rise Positive  vinit=0  OutDataTypeStr=boolean
  Relational Operator : RelationalOperator  OutDataTypeStr=boolean  RndMeth=Simplest
  Scope : Scope
  Scope1 : Scope
  Series RLC Branch : powerlib/Elements/Series RLC Branch  LConnTagsString=__new0  RConnTagsString=__new0  BranchType=R  Resistance=R52  Inductance=1e-3  SetiL0=off  InitialCurrent=0  Capacitance=1e-6  Setx0=off  InitialVoltage=0  Measurements=None
      settings: SourceProductName=Simscape Electrical
  Switch1 : Switch  Criteria=u2 > Threshold
  Thyristor : powerlib/Power Electronics/Thyristor  Ron=0.001  Lon=0  Vf=0.8  IC=0  Rs=500  Cs=250e-9  Measurements=off
      settings: SourceProductName=Simscape Electrical
  To Workspace1 : ToWorkspace  VariableName=corrente_tiristor_r_2  SampleTime=-1
  To Workspace4 : ToWorkspace  VariableName=tensao_tiristor_r_2  SampleTime=-1
  V_Load : powerlib/Measurements/Voltage Measurement  PhasorSimulation=off  OutputType=Complex  PSBequivalent=0
      settings: SourceProductName=Simscape Electrical
  V_Load1 : powerlib/Measurements/Voltage Measurement  PhasorSimulation=off  OutputType=Complex  PSBequivalent=0
      settings: SourceProductName=Simscape Electrical
  i_Load : powerlib/Measurements/Current Measurement  Tag=PoWeRsYsTeMmEaSuReMeNt  PhasorSimulation=off  OutputType=Magnitude  PSBequivalent=0
      settings: SourceProductName=Simscape Electrical
  Conn1 : PMIOPort  Side=Left
  Conn2 : PMIOPort  Port=2  Side=Left
  wires:
  Constant3/1 -> Switch1/3
  Constant2/1 -> Switch1/1
  Constant1/1 -> Relational Operator/2
  Relational Operator/1 -> Detect Rise Positive/1
  i_Load/1 -> To Workspace1/1, Scope1/1
  Detect Rise Positive/1 -> Switch1/2
  V_Load1/1 -> Relational Operator/1
  V_Load/1 -> Scope/1, To Workspace4/1
  Switch1/1 -> Thyristor/1
  connections:
  V_Load/LConn1 -- Thyristor/RConn1 -- Series RLC Branch/LConn1
  Conn1/RConn1 -- V_Load1/LConn1 -- i_Load/LConn1
  i_Load/RConn1 -- Thyristor/LConn1
  V_Load/LConn2 -- Series RLC Branch/RConn1 -- Conn2/RConn1 -- V_Load1/LConn2

== system Sim_Induct_Harmon/THYRISTOR_R_3 ==
  note: LOAD
  Constant1 : Constant  Value=Valpha5
  Constant2 : Constant  Value=5
  Constant3 : Constant  Value=0
  Detect Rise Positive : simulink/Logic and Bit Operations/Detect Rise Positive  vinit=0  OutDataTypeStr=boolean
  Relational Operator : RelationalOperator  OutDataTypeStr=boolean  RndMeth=Simplest
  Scope : Scope
  Scope1 : Scope
  Series RLC Branch : powerlib/Elements/Series RLC Branch  LConnTagsString=__new0  RConnTagsString=__new0  BranchType=R  Resistance=R53  Inductance=1e-3  SetiL0=off  InitialCurrent=0  Capacitance=1e-6  Setx0=off  InitialVoltage=0  Measurements=None
      settings: SourceProductName=Simscape Electrical
  Switch1 : Switch  Criteria=u2 > Threshold
  Thyristor : powerlib/Power Electronics/Thyristor  Ron=0.001  Lon=0  Vf=0.8  IC=0  Rs=500  Cs=250e-9  Measurements=off
      settings: SourceProductName=Simscape Electrical
  To Workspace1 : ToWorkspace  VariableName=corrente_tiristor_r_3  SampleTime=-1
  To Workspace4 : ToWorkspace  VariableName=tensao_tiristor_r_3  SampleTime=-1
  V_Load : powerlib/Measurements/Voltage Measurement  PhasorSimulation=off  OutputType=Complex  PSBequivalent=0
      settings: SourceProductName=Simscape Electrical
  V_Load1 : powerlib/Measurements/Voltage Measurement  PhasorSimulation=off  OutputType=Complex  PSBequivalent=0
      settings: SourceProductName=Simscape Electrical
  i_Load : powerlib/Measurements/Current Measurement  Tag=PoWeRsYsTeMmEaSuReMeNt  PhasorSimulation=off  OutputType=Magnitude  PSBequivalent=0
      settings: SourceProductName=Simscape Electrical
  Conn1 : PMIOPort  Side=Left
  Conn2 : PMIOPort  Port=2  Side=Left
  wires:
  Constant3/1 -> Switch1/3
  Constant2/1 -> Switch1/1
  Constant1/1 -> Relational Operator/2
  Relational Operator/1 -> Detect Rise Positive/1
  i_Load/1 -> To Workspace1/1, Scope1/1
  Detect Rise Positive/1 -> Switch1/2
  V_Load1/1 -> Relational Operator/1
  V_Load/1 -> Scope/1, To Workspace4/1
  Switch1/1 -> Thyristor/1
  connections:
  V_Load/LConn1 -- Thyristor/RConn1 -- Series RLC Branch/LConn1
  Conn1/RConn1 -- V_Load1/LConn1 -- i_Load/LConn1
  i_Load/RConn1 -- Thyristor/LConn1
  V_Load/LConn2 -- Series RLC Branch/RConn1 -- Conn2/RConn1 -- V_Load1/LConn2

== system Sim_Induct_Harmon/THYRISTOR_R_4 ==
  note: LOAD
  Constant1 : Constant  Value=Valpha5
  Constant2 : Constant  Value=5
  Constant3 : Constant  Value=0
  Detect Rise Positive : simulink/Logic and Bit Operations/Detect Rise Positive  vinit=0  OutDataTypeStr=boolean
  Relational Operator : RelationalOperator  OutDataTypeStr=boolean  RndMeth=Simplest
  Scope : Scope
  Scope1 : Scope
  Series RLC Branch : powerlib/Elements/Series RLC Branch  LConnTagsString=__new0  RConnTagsString=__new0  BranchType=R  Resistance=R54  Inductance=1e-3  SetiL0=off  InitialCurrent=0  Capacitance=1e-6  Setx0=off  InitialVoltage=0  Measurements=None
      settings: SourceProductName=Simscape Electrical
  Switch1 : Switch  Criteria=u2 > Threshold
  Thyristor : powerlib/Power Electronics/Thyristor  Ron=0.001  Lon=0  Vf=0.8  IC=0  Rs=500  Cs=250e-9  Measurements=off
      settings: SourceProductName=Simscape Electrical
  To Workspace1 : ToWorkspace  VariableName=corrente_tiristor_r_4  SampleTime=-1
  To Workspace4 : ToWorkspace  VariableName=tensao_tiristor_r_4  SampleTime=-1
  V_Load : powerlib/Measurements/Voltage Measurement  PhasorSimulation=off  OutputType=Complex  PSBequivalent=0
      settings: SourceProductName=Simscape Electrical
  V_Load1 : powerlib/Measurements/Voltage Measurement  PhasorSimulation=off  OutputType=Complex  PSBequivalent=0
      settings: SourceProductName=Simscape Electrical
  i_Load : powerlib/Measurements/Current Measurement  Tag=PoWeRsYsTeMmEaSuReMeNt  PhasorSimulation=off  OutputType=Magnitude  PSBequivalent=0
      settings: SourceProductName=Simscape Electrical
  Conn1 : PMIOPort  Side=Left
  Conn2 : PMIOPort  Port=2  Side=Left
  wires:
  Constant3/1 -> Switch1/3
  Constant2/1 -> Switch1/1
  Constant1/1 -> Relational Operator/2
  Relational Operator/1 -> Detect Rise Positive/1
  i_Load/1 -> To Workspace1/1, Scope1/1
  Detect Rise Positive/1 -> Switch1/2
  V_Load1/1 -> Relational Operator/1
  V_Load/1 -> Scope/1, To Workspace4/1
  Switch1/1 -> Thyristor/1
  connections:
  V_Load/LConn1 -- Thyristor/RConn1 -- Series RLC Branch/LConn1
  Conn1/RConn1 -- V_Load1/LConn1 -- i_Load/LConn1
  i_Load/RConn1 -- Thyristor/LConn1
  V_Load/LConn2 -- Series RLC Branch/RConn1 -- Conn2/RConn1 -- V_Load1/LConn2

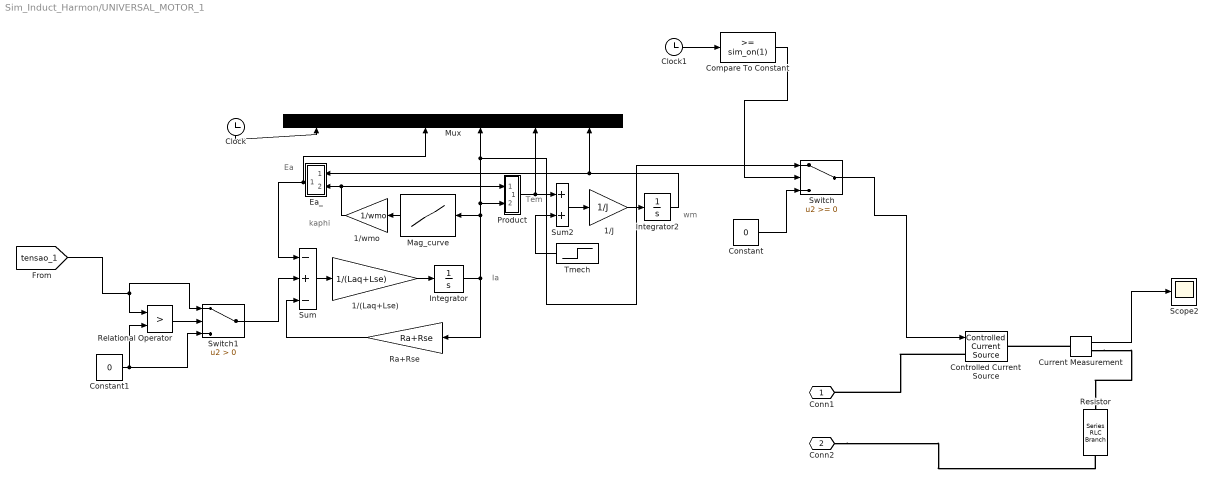
== system Sim_Induct_Harmon/UNIVERSAL_MOTOR_1 ==
  note: kaphi
  note: Tem
  note: Ea
  note: wm
  note: Ia
  1/(Laq+Lse) : Gain  Gain=1/(Laq+Lse)  SaturateOnIntegerOverflow=on  OutDataTypeStr=Inherit: Same as input  ParamDataTypeStr=Inherit: Same as input
  1/J : Gain  Gain=1/J  SaturateOnIntegerOverflow=on  OutDataTypeStr=Inherit: Same as input  ParamDataTypeStr=Inherit: Same as input
  1/wmo : Gain  Gain=1/wmo  SaturateOnIntegerOverflow=on  OutDataTypeStr=Inherit: Same as input  ParamDataTypeStr=Inherit: Same as input
  Clock : Clock
  Clock1 : Clock
  Compare To Constant : simulink/Logic and Bit Operations/Compare To Constant  relop=>=  const=sim_on(1)  OutDataTypeStr=boolean
  Constant : Constant  Value=0
  Constant1 : Constant  Value=0
  Controlled Current Source : powerlib/Electrical Sources/Controlled Current Source  Initialize=on  Source_Type=AC  Amplitude=0  Phase=0  Frequency=0  Measurements=None
      settings: SourceProductName=Simscape Electrical
  Current Measurement : powerlib/Measurements/Current Measurement  PhasorSimulation=off  OutputType=Complex  PSBequivalent=0
      settings: SourceProductName=Simscape Electrical
  Ea_ : Subsystem  mask(Dot Product){}
      mask help:
      | Inner (dot) product.
      | y=sum(u1.*u2)
      mask Help: Computes the inner (dot) product of the inputs: sum(u1.*u2).  The inputs are vectors of the same length. Output is a scalar.
      mask Display: disp('.\n')
  Integrator : Integrator
  Integrator2 : Integrator  InitialCondition=wm0
  Mag_curve : Lookup  InputValues=SEIP4  Table=SEVP4  SaturateOnIntegerOverflow=on
  Mux : Mux  Inputs=6
  Product : Subsystem  mask(Dot Product){}
      mask help:
      | Inner (dot) product.
      | y=sum(u1.*u2)
      mask Help: Computes the inner (dot) product of the inputs: sum(u1.*u2).  The inputs are vectors of the same length. Output is a scalar.
      mask Display: disp('.\n')
  Ra+Rse : Gain  Gain=Ra+Rse  SaturateOnIntegerOverflow=on  OutDataTypeStr=Inherit: Same as input  ParamDataTypeStr=Inherit: Same as input
  Relational Operator : RelationalOperator  Operator=>  OutDataTypeStr=boolean  RndMeth=Simplest
  Resistor : powerlib/Elements/Series RLC Branch  LConnTagsString=__new0  RConnTagsString=__new0  BranchType=R  Resistance=1e-15  Inductance=1e-3  SetiL0=off  InitialCurrent=0  Capacitance=1e-6  Setx0=off  InitialVoltage=0  Measurements=None
      settings: SourceProductName=Simscape Electrical
  Scope2 : Scope
  Sum : Sum  Inputs=-+-  SaturateOnIntegerOverflow=on  InputSameDT=on  OutDataTypeStr=Inherit: Same as first input
  Sum2 : Sum  SaturateOnIntegerOverflow=on  InputSameDT=on  OutDataTypeStr=Inherit: Same as first input
  Switch : Switch
  Switch1 : Switch  Criteria=u2 > Threshold
  Tmech : Step  Time=0  Before=-0.8  After=2
  Conn1 : PMIOPort  Side=Left
  Conn2 : PMIOPort  Port=2  Side=Left
  wires:
  Ra+Rse/1 -> Sum/3
  1/J/1 -> Integrator2/1
  1/wmo/1 -> Ea_/2(in_2), Product/1(in_1)
  Current Measurement/1 -> Scope2/1
  Mag_curve/1 -> 1/wmo/1
  Sum/1 -> 1/(Laq+Lse)/1
  Sum2/1 -> 1/J/1
  1/(Laq+Lse)/1 -> Integrator/1
  Ea_/1(out_1) -> Mux/3, Sum/1
  Integrator2/1 -> Mux/6, Ea_/1(in_1)
  Tmech/1 -> Sum2/2
  Integrator/1 -> Switch/1, Mux/4, Product/2(in_2), Mag_curve/1, Ra+Rse/1
  Clock/1 -> Mux/1
  Product/1(out_1) -> Mux/5, Sum2/1
  Constant/1 -> Switch/3
  Compare To Constant/1 -> Switch/2
  Clock1/1 -> Compare To Constant/1
  Switch/1 -> Controlled Current Source/1
  Relational Operator/1 -> Switch1/2
  Constant1/1 -> Relational Operator/2, Switch1/3
  Switch1/1 -> Sum/2
  [tensao_1] -> Relational Operator/1, Switch1/1
  connections:
  Conn2/RConn1 -- Resistor/RConn1
  Controlled Current Source/LConn1 -- Conn1/RConn1
  Current Measurement/LConn1 -- Controlled Current Source/RConn1
  Current Measurement/RConn1 -- Resistor/LConn1
